simulink library "pbbs"  (Simulink 8.1)
settings: Solver=ode1  StartTime=0.0  StopTime=Inf  FixedStep=0.001  RelTol=1e-3
PostLoadFcn:
  | , if any(exist('dsrtsu_mdlpostloadfcn', 'file') == [2, 3, 6]), try dsrtsu_mdlpostloadfcn('Execute', bdroot); catch fprintf('Error in PostLoadFcn (dsrtsu_mdlpostloadfcn) for model "%s":\n %s\n', bdroot, lasterr); end, end,
libraries: ebdc x1, frdc x1, ntbdc x1, tbdc x1
settings Model: DSRTSU_INTERNAL_RTI_VER=450  DSRTSU_INTERNAL_RTI_TYPE=rti1401  RTICANMMDATA=struct('GeneralSetupData',struct('modelroot','D:\PROJECTS\HAITEC\TAIWAN_HAITEC_SVN\branches\Model_with_Distance_trigger\AdasDragon\software\sw_development\arch\app\jud','generalsettings',struct('filesettings',struct('destfolder',struct('Name','RTICANMM_FILES','Check',1),'buildfolder',struct('Name','.','Check',1),'AbsDestfolder',struct('Name','D:\PROJECTS\HAITEC\TAIWAN_HAITEC_SVN\branches\Model_with_Distance_trigger\AdasDragon\software\sw_development\arch\app\jud\RTICANMM_FILES'),'AbsBuildfolder',struct('Name','D:\PROJECTS\HAITEC\TAIWAN_HAITEC_SVN\branches\Model_with_Distance_trigger\AdasDragon\software\sw_development\arch\app\jud'))),'options',struct('addpaths',1,'rmpaths',1,'addtrcexclusion',logical(1),'cannavigator',struct('checkmonitoring',0),'show_usrtrc',0,'use_usrtrc',0),'advanced',struct('options',[1 1 1 1 1 1 1 1 1 1 1 1 1 1 1 1 1 1 1 1 1 1 1 1 1 1 1 1 1 1 1 1 1 1 1 1 1 1 1 1 1 1 1 1 1 1 1 1 1 1 1 1 1 1 1 1 1 1 1 1 1 1 1 1 1 1 1 1 1 1 1 1 1 1 1 1 1 1 1 1 1 1 1 1 1 1 1 1 1 1 1 1 1 1 1 1 1 1 1 1]),'MPSetup',{{}},'modelname','pbbs','block','pbbs'))  DSRTSU_INTERNAL_RTIFPGA=40  Creator=tescamilla  LastModifiedBy=aitor

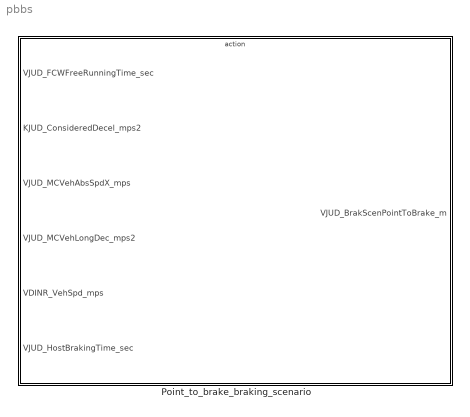
== system pbbs ==
  Point_to_brake_braking_scenario : Subsystem

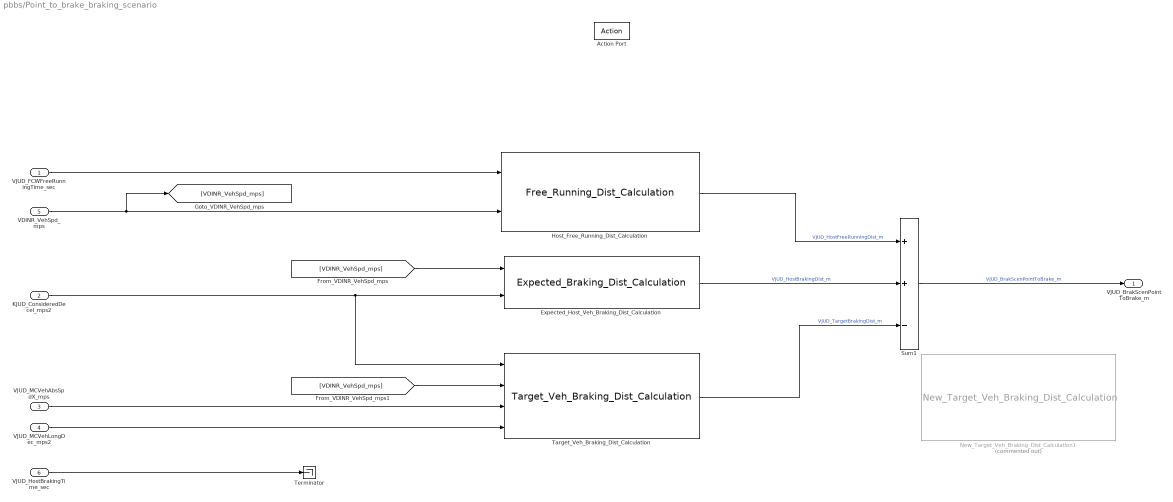
== system pbbs/Point_to_brake_braking_scenario ==
  VJUD_FCWFreeRunningTime_sec : Inport
  KJUD_ConsideredDecel_mps2 : Inport  Port=2
  VJUD_MCVehAbsSpdX_mps : Inport  Port=3
  VJUD_MCVehLongDec_mps2 : Inport  Port=4
  VDINR_VehSpd_mps : Inport  Port=5
  VJUD_HostBrakingTime_sec : Inport  Port=6
  Action Port : ActionPort
  Expected_Host_Veh_Braking_Dist_Calculation : ebdc/Expected_Braking_Dist_Calculation
  Host_Free_Running_Dist_Calculation : frdc/Free_Running_Dist_Calculation
  New_Target_Veh_Braking_Dist_Calculation1 : ntbdc/New_Target_Veh_Braking_Dist_Calculation  Commented=on
  Sum1 : Sum  Inputs=++-
  Target_Veh_Braking_Dist_Calculation : tbdc/Target_Veh_Braking_Dist_Calculation
  Terminator : Terminator
  VJUD_BrakScenPointToBrake_m : Outport
  wires:
  KJUD_ConsideredDecel_mps2/1 -> Target_Veh_Braking_Dist_Calculation/1, Expected_Host_Veh_Braking_Dist_Calculation/2
  VJUD_MCVehLongDec_mps2/1 -> Target_Veh_Braking_Dist_Calculation/4
  VJUD_FCWFreeRunningTime_sec/1 -> Host_Free_Running_Dist_Calculation/1
  Host_Free_Running_Dist_Calculation/1 -> Sum1/1  "VJUD_HostFreeRunningDist_m"
  Expected_Host_Veh_Braking_Dist_Calculation/1 -> Sum1/2  "VJUD_HostBrakingDist_m"
  VJUD_MCVehAbsSpdX_mps/1 -> Target_Veh_Braking_Dist_Calculation/3
  Target_Veh_Braking_Dist_Calculation/1 -> Sum1/3  "VJUD_TargetBrakingDist_m"
  VDINR_VehSpd_mps/1 -> [VDINR_VehSpd_mps], Host_Free_Running_Dist_Calculation/2
  Sum1/1 -> VJUD_BrakScenPointToBrake_m/1  "VJUD_BrakScenPointToBrake_m"
  [VDINR_VehSpd_mps] -> Expected_Host_Veh_Braking_Dist_Calculation/1
  VJUD_HostBrakingTime_sec/1 -> Terminator/1
  [VDINR_VehSpd_mps] -> Target_Veh_Braking_Dist_Calculation/2
